simulink model "tank_with_fuzzy"  (R2017a)
settings: Solver=FixedStepAuto  StartTime=0.0  StopTime=400  FixedStep=0.2  RelTol=1e-3  EnableMultiTasking=on
libraries: fuzblock x1, powerlib_meascontrol x1
settings Model: Creator=MiniElite705g2  LastModifiedBy=hdg19
settings DataIOCC: LimitDataPoints=on  SaveFormat=Array  SignalLoggingSaveFormat=ModelDataLogs
settings OptimizationCC: InitFltsAndDblsToZero=on  LifeSpan=inf
settings DebuggingCC: SaveWithParameterizedLinksMsg=none  UnderspecifiedInitializationDetection=Classic  MergeDetectMultiDrivingBlocksExec=none  SignalResolutionControl=TryResolveAllWithWarning  SolverPrmCheckMsg=warning  MultiTaskDSMMsg=warning  MultiTaskCondExecSysMsg=none  SFUnexpectedBacktrackingDiag=warning  SFNoUnconditionalDefaultTransitionDiag=warning  SFExecutionAtInitializationDiag=none
settings HardwareCC: ProdBitPerPointer=32  ProdBitPerSizeT=32  ProdBitPerPtrDiffT=32  ProdLargestAtomicFloat=None  ProdIntDivRoundTo=Undefined  ProdEndianess=Unspecified  ProdWordSize=32  ProdHWDeviceType=32-bit Generic
settings ModelReferenceCC: PropagateSignalLabelsOutOfModel=off
settings GRTTargetCC: TargetFcnLib=ansi_tfl_tmw.mat  TargetLangStandard=C89/C90 (ANSI)  GeneratePreprocessorConditionals=Disable all  CombineOutputUpdateFcns=off  GRTInterface=on
settings ConfigComp: CovMetricSettings=dw  CovHtmlReporting=on  CovSaveCumulativeToWorkspaceVar=on  CovSaveSingleToWorkspaceVar=on  CovExternalEMLEnable=off  CovSFcnEnable=off

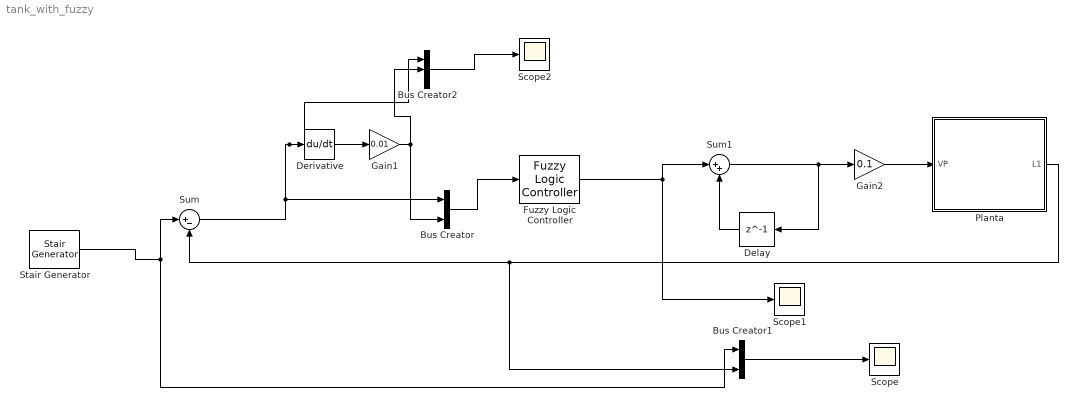
== system tank_with_fuzzy ==
  Bus Creator : BusCreator  Inputs=2
  Bus Creator1 : BusCreator  Inputs=2
  Bus Creator2 : BusCreator  Inputs=3
  Delay : Delay  DelayLength=1  InitialCondition=0
  Derivative : Derivative
  Fuzzy Logic Controller : fuzblock/Fuzzy Logic  Controller  fis='fuzzy_tank.fis'
  Gain1 : Gain  Gain=0.01
  Gain2 : Gain  Gain=0.1
  Planta : Subsystem  mask(TANKS){a1=media, a2=media}
      mask prompts: a1 "Area do orificio de T1"; a2 "Area do orificio de T2"
      mask help: Esse e o modelo dos tanks acoplados
      mask Help: E uma pena
      mask TypeOptions a1: pequena | media | grande
      mask TypeOptions a2: pequena | media | grande
  Scope : Scope
  Scope1 : Scope
  Scope2 : Scope
  Stair Generator : powerlib_meascontrol/Pulse & Signal Generators/Stair Generator  t=[0, 200]  e=[14, 10]  Ts=0
      settings: SourceProductName=Simscape Power Systems
  Sum : Sum  Inputs=|+-
  Sum1 : Sum  Inputs=|++
  wires:
  Stair Generator/1 -> Sum/1, Bus Creator1/1
  Planta/1(L1) -> Bus Creator1/2, Sum/2
  Derivative/1 -> Gain1/1
  Bus Creator/1 -> Fuzzy Logic Controller/1
  Bus Creator1/1 -> Scope/1
  Bus Creator2/1 -> Scope2/1
  Sum/1 -> Bus Creator2/1, Derivative/1, Bus Creator/1
  Gain1/1 -> Bus Creator/2, Bus Creator2/2
  Sum1/1 -> Gain2/1, Delay/1
  Delay/1 -> Sum1/2
  Fuzzy Logic Controller/1 -> Sum1/1, Scope1/1
  Gain2/1 -> Planta/1(VP)

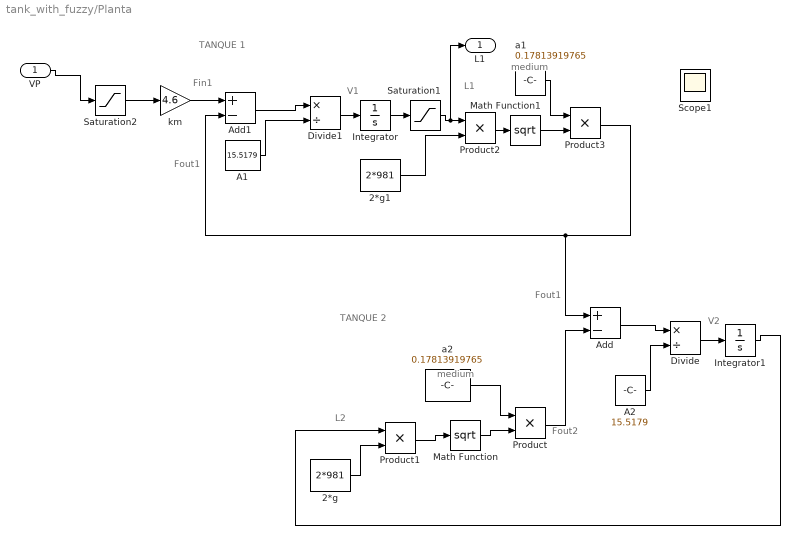
== system tank_with_fuzzy/Planta ==
  note: Fin1
  note: L2
  note: Fout1
  note: Fout2
  note: L1
  note: Fout1
  note: TANQUE 2
  note: TANQUE 1
  note: medium
  note: medium
  note: V1
  note: V2
  VP : Inport
  2*g : Constant  Value=2*981
  2*g1 : Constant  Value=2*981
  A1 : Constant  Value=15.5179
  A2 : Constant  Value=15.5179
  Add : Sum  Inputs=+-
  Add1 : Sum  Inputs=+-
  Divide : Product  Inputs=*/
  Divide1 : Product  Inputs=*/
  Integrator : Integrator
  Integrator1 : Integrator  UpperSaturationLimit=30  LowerSaturationLimit=-30
  Math Function : Math  Operator=sqrt  SaturateOnIntegerOverflow=on
  Math Function1 : Math  Operator=sqrt  SaturateOnIntegerOverflow=on
  Product{,1..3} (4 alike) : Product  RndMeth=Zero
  Saturation1 : Saturate  UpperLimit=30  LowerLimit=0
  Saturation2 : Saturate  UpperLimit=15  LowerLimit=-15
  Scope1 : Scope
  a1 : Constant  Value=0.17813919765
  a2 : Constant  Value=0.17813919765
  km : Gain  Gain=4.6
  L1 : Outport
  wires:
  VP/1 -> Saturation2/1
  2*g/1 -> Product1/2
  Product1/1 -> Math Function/1
  a2/1 -> Product/1
  Math Function/1 -> Product/2
  Product/1 -> Add/2
  Add/1 -> Divide/1
  A2/1 -> Divide/2
  Divide/1 -> Integrator1/1
  Integrator1/1 -> Product1/1
  Add1/1 -> Divide1/1
  A1/1 -> Divide1/2
  Divide1/1 -> Integrator/1
  2*g1/1 -> Product2/2
  Product2/1 -> Math Function1/1
  Math Function1/1 -> Product3/2
  a1/1 -> Product3/1
  Product3/1 -> Add1/2, Add/1
  km/1 -> Add1/1
  Integrator/1 -> Saturation1/1
  Saturation1/1 -> Product2/1, L1/1
  Saturation2/1 -> km/1
